simulink subsystem "distance3d"  (R2023a)
settings: Solver=VariableStepAuto  StartTime=0.0  StopTime=10.0  RelTol=1e-3
settings Model: Creator=bjmyn  LastModifiedBy=bjmyn

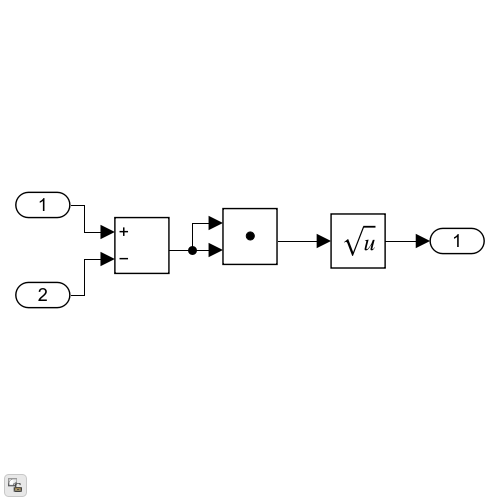
[thumbnail: Simulink's stored preview of the top-level diagram]
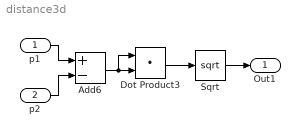
== system distance3d ==
  p1 : Inport
  p2 : Inport  Port=2
  Add6 : Sum  Inputs=+-
  Dot Product3 : DotProduct  OutDataTypeStr=Inherit: Inherit via internal rule
  Sqrt : Sqrt
  Out1 : Outport
  wires:
  Sqrt/1 -> Out1/1
  p2/1 -> Add6/2
  p1/1 -> Add6/1
  Add6/1 -> Dot Product3/1, Dot Product3/2
  Dot Product3/1 -> Sqrt/1
